simulink model "FlywheelSimscapeWithSensors"  (R2016a)
settings: Solver=VariableStepAuto  StartTime=0.0  StopTime=1000  RelTol=1e-3
undefined symbols (not defined in the file): sigbuilder_block
libraries: fl_lib x14, nesl_utility x8
settings Model: Creator=chiavazzo  LastModifiedBy=chiavazzo

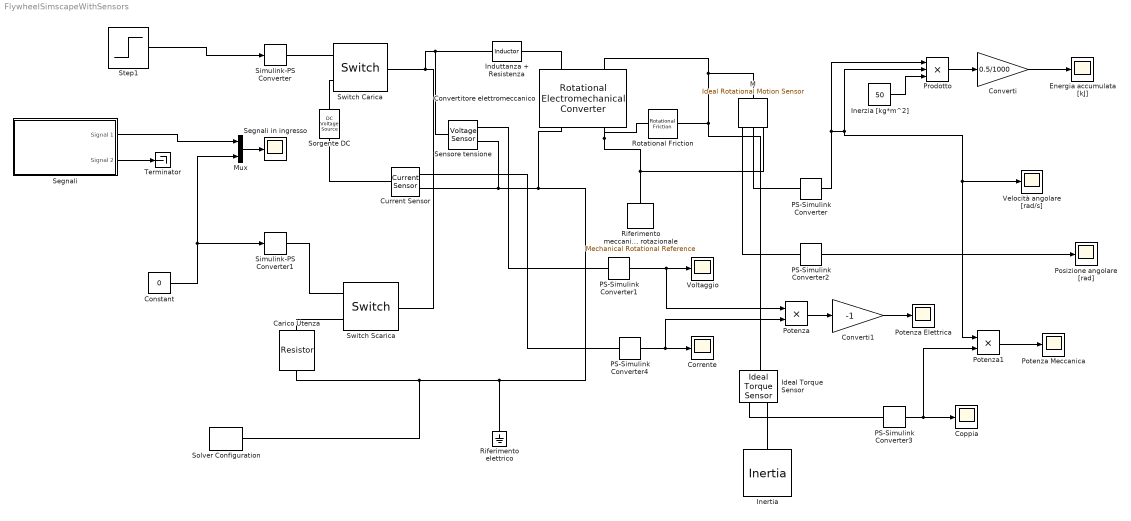
== system FlywheelSimscapeWithSensors ==
  " M" : fl_lib/Mechanical/Mechanical Sensors/Ideal Rotational Motion Sensor  offset=0 rad
  Carico Utenza : fl_lib/Electrical/Electrical Elements/Resistor  R=3 Ohm  i_specify=off  i_priority=None  i=0 A  v_specify=off  v_priority=None  v=0 V
  Constant : Constant  Value=0
  Converti : Gain  Gain=0.5/1000
  Converti1 : Gain  Gain=-1
  Convertitore elettromeccanico : fl_lib/Electrical/Electrical Elements/Rotational Electromechanical Converter  K=0.23 V/(rad/s)  i_specify=off  i_priority=None  i=0 A  v_specify=off  v_priority=None  v=0 V  t_specify=off  t_priority=None  t=0 N*m  w_specify=off  w_priority=None  w=0 rad/s
  Coppia : Scope
  Corrente : Scope
  Current Sensor : fl_lib/Electrical/Electrical Sensors/Current Sensor
  Energia accumulata [kJ] : Scope
  Ideal Torque Sensor : fl_lib/Mechanical/Mechanical Sensors/Ideal Torque Sensor
  Induttanza + Resistenza : fl_lib/Electrical/Electrical Elements/Inductor  l=5e-3 H  r=0.5 Ohm  g=1e-9 1/Ohm  i_specify=off  i_priority=None  i=0 A  v_specify=off  v_priority=None  v=0 V  i_L_specify=off  i_L_priority=High  i_L=0 A
  Inertia : fl_lib/Mechanical/Rotational Elements/Inertia  inertia=50 kg*m^2  w_specify=on  w_priority=High  w=0 rad/s  t_specify=off  t_priority=None  t=0 N*m
  Inerzia [kg*m^2] : Constant  Value=50
  Mux : Mux  Inputs=2
  PS-Simulink Converter{,1..4} (5 alike) : nesl_utility/PS-Simulink Converter  PhysicalDomain=network_engine_domain  SubClassName=ps_output  LeftPortType=input  RightPortType=output  PseudoPeriodic=off  Frequencies=[]  Unit=1  AffineConversion=off
  Posizione angolare [rad] : Scope
  Potenza : Product
  Potenza Elettrica : Scope
  Potenza Meccanica : Scope
  Potenza1 : Product
  "Prodotto " : Product  Inputs=3
  Riferimento meccanico rotazionale : fl_lib/Mechanical/Rotational Elements/Mechanical Rotational Reference
  Riferimento elettrico : fl_lib/Electrical/Electrical Elements/Electrical Reference
  Rotational Friction : fl_lib/Mechanical/Rotational Elements/Rotational Friction  brkwy_trq=25e-3 N*m  Col_trq=20e-3 N*m  visc_coef=0.01 N*m/(rad/s)  trans_coef=10 s/rad  vel_thr=1e-4 rad/s  w_specify=off  w_priority=None  w=0 rad/s  t_specify=off  t_priority=None  t=0 N*m
  Segnali : Subsystem  Tag=STV Subsys  LoadFcn=sigbuilder_block('load');  StartFcn=sigbuilder_block('start');  StopFcn=sigbuilder_block('stop');  ClipboardFcn=sigbuilder_block('clipboard');  mask(Sigbuilder block){}
      mask help: Simulink:masks:SigbuilderBlock_MD
      mask init:
      | if ~strcmp(get_param(bdroot(gcbh),'SimulationStatus'),'stopped') tuvar = sigbuilder_block('maskInit'); end
      settings: CopyFcn=sigbuilder_block('copy');  DeleteFcn=sigbuilder_block('delete');  ModelCloseFcn=sigbuilder_block('modelClose');  PreSaveFcn=sigbuilder_block('preSave');  PauseFcn=sigbuilder_block('pause');  ContinueFcn=sigbuilder_block('continue');  NameChangeFcn=sigbuilder_block('namechange');  OpenFcn=sigbuilder_block('open',[124.5 40.5 738 329.5 ]);  CloseFcn=sigbuilder_block('close');
      mask Display: plot(0, 0, 100, 100,[2, 2, 32, 32, 2], [68, 8, 8, 68, 68],[32, 2], [38, 38], [32, 19, 2],[53, 60, 44], [32, 17, 17, 2],[16, 16, 31, 31]);txt = getActiveGroup(gcbh);text(2, 100, txt,'verticalAlignment', 'top');
  Segnali in ingresso : Scope
  Sensore tensione : fl_lib/Electrical/Electrical Sensors/Voltage Sensor
  Simulink-PS Converter : nesl_utility/Simulink-PS Converter  PhysicalDomain=network_engine_domain  SubClassName=ps_input  LeftPortType=input  RightPortType=output  PseudoPeriodic=off  Frequencies=[]  NoiseDistribution=none  NoiseParameters=[]  Unit=1  AffineConversion=off  InputFiltering=off  SimscapeFilterOrder=1  InputFilterTimeConstant=0.001  UdotUserProvided=1
  Simulink-PS Converter1 : nesl_utility/Simulink-PS Converter  PhysicalDomain=network_engine_domain  SubClassName=ps_input  LeftPortType=input  RightPortType=output  PseudoPeriodic=off  Frequencies=[]  NoiseDistribution=none  NoiseParameters=[]  Unit=1  AffineConversion=off  InputFiltering=off  SimscapeFilterOrder=1  InputFilterTimeConstant=0.001  UdotUserProvided=1
  Solver Configuration : nesl_utility/Solver Configuration  PhysicalDomain=network_engine_domain  SubClassName=solver  LeftPortType=input  RightPortType=generic  Accelerate=off  Tones=[]  Harmonics=[]  SimulateNoise=off  Profile=off  UseLocalSampling=off  EnableSwitchedLinearOptims=on  FrequencyDomain=off  UseCCode=off  RelTol=0.001  AbsTol=1e-06  MinStep=1e-09  ToWorkspace=off  RevertToSquareIcSolve=off  NumHomotopyIterations=100  PhasorMode=off  PhasorModeNumHarmonics=1  OverrideAbsTol=off  DoDC=off  ResidualTolerance=1e-09  UseLocalSolver=on  LocalSolverChoice=NE_BACKWARD_EULER_ADVANCER  LocalSolverSampleTime=0.001  DoFixedCost=on  MaxNonlinIter=3  MaxModeIter=2  LinearAlgebra=Sparse  DelaysMemoryBudget=1024  AutomaticFiltering=on  FilteringTimeConstant=0.001
  Sorgente DC : fl_lib/Electrical/Electrical Sources/DC Voltage Source  v0=50 V
  Step1 : Step  Time=10  SampleTime=0
  Switch Carica : fl_lib/Electrical/Electrical Elements/Switch  R_closed=0.01 Ohm  G_open=1e-8 1/Ohm  Threshold=1e-3  i_specify=off  i_priority=None  i=0 A  v_specify=off  v_priority=None  v=0 V
  Switch Scarica : fl_lib/Electrical/Electrical Elements/Switch  R_closed=0.01 Ohm  G_open=1e-8 1/Ohm  Threshold=1e-3  i_specify=off  i_priority=None  i=0 A  v_specify=off  v_priority=None  v=0 V
  Terminator : Terminator
  Velocità angolare [rad/s] : Scope
  Voltaggio : Scope
  wires:
  PS-Simulink Converter/1 -> "Prodotto "/1, "Prodotto "/2, Potenza1/1, Velocità angolare [rad/s]/1
  PS-Simulink Converter2/1 -> Posizione angolare [rad]/1
  PS-Simulink Converter1/1 -> Potenza/1, Voltaggio/1
  "Prodotto "/1 -> Converti/1
  Inerzia [kg*m^2]/1 -> "Prodotto "/3
  Converti/1 -> Energia accumulata [kJ]/1
  Mux/1 -> Segnali in ingresso/1
  Constant/1 -> Mux/2, Simulink-PS Converter1/1
  Segnali/2(Signal 2) -> Terminator/1
  Step1/1 -> Simulink-PS Converter/1
  Segnali/1(Signal 1) -> Mux/1
  PS-Simulink Converter3/1 -> Potenza1/2, Coppia/1
  PS-Simulink Converter4/1 -> Potenza/2, Corrente/1
  Potenza/1 -> Converti1/1
  Potenza1/1 -> Potenza Meccanica/1
  Converti1/1 -> Potenza Elettrica/1
  connections:
  Induttanza + Resistenza/RConn1 -- Convertitore elettromeccanico/LConn1
  Convertitore elettromeccanico/RConn2 -- Rotational Friction/LConn1 -- " M"/RConn1 -- Riferimento meccanico rotazionale/LConn1
  " M"/RConn2 -- PS-Simulink Converter/LConn1
  " M"/RConn3 -- PS-Simulink Converter2/LConn1
  Sensore tensione/RConn1 -- PS-Simulink Converter1/LConn1
  Sorgente DC/LConn1 -- Switch Carica/RConn2
  Simulink-PS Converter/RConn1 -- Switch Carica/RConn1
  Carico Utenza/LConn1 -- Switch Scarica/RConn2
  Simulink-PS Converter1/RConn1 -- Switch Scarica/RConn1
  Solver Configuration/RConn1 -- Carico Utenza/RConn1 -- Riferimento elettrico/LConn1 -- Current Sensor/RConn2 -- Sensore tensione/RConn2 -- Convertitore elettromeccanico/RConn1
  Convertitore elettromeccanico/LConn2 -- Ideal Torque Sensor/LConn1 -- Rotational Friction/RConn1 -- " M"/LConn1
  Switch Carica/LConn1 -- Switch Scarica/LConn1 -- Sensore tensione/LConn1 -- Induttanza + Resistenza/LConn1
  PS-Simulink Converter4/LConn1 -- Current Sensor/RConn1
  Ideal Torque Sensor/RConn1 -- Inertia/LConn1
  Ideal Torque Sensor/RConn2 -- PS-Simulink Converter3/LConn1
  Current Sensor/LConn1 -- Sorgente DC/RConn1

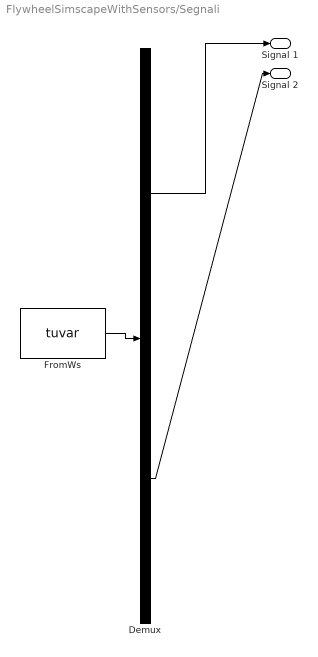
== system FlywheelSimscapeWithSensors/Segnali ==
  Demux : Demux  Tag=STV Demux  Outputs=2
  FromWs : FromWorkspace  Tag=STV FromWs  VariableName=tuvar  SampleTime=0
      SigBuilderData=|
      | common.afterFinalStr = 'Extrapolate'
      | common.sampleTime = 0
      | dataSet.timeRange = [0 15]
      | dataSet.name = 'Group 1'
      | sbobj.Groups.Name = 'Group 1'
      | sbobj.Groups.Signals(1).Name = 'Signal 1'
      | sbobj.Groups.Signals(1).XData = [0 4 6 6 15]
      | sbobj.Groups.Signals(1).YData = [1 1 1 0 0]
      | sbobj.Groups.Signals(2).Name = 'Signal 2'
      | sbobj.Groups.Signals(2).XData = [0 1 1.5 2 2.5 3 3.5 4 4.5 5 5.5 6 6.5 7 7.5 8 8.5 9 9.5 10 10 11 11.5 12 12.5 14.5 14.5 15]
      | sbobj.Groups.Signals(2).YData = [0 1.22464679915e-16 0 0 0 1.22464679915e-16 0 0 0 1.22464679915e-16 0 0 0 1.22464679915e-16 0 0 0 1.22464679915e-16 0 0 1 1 1 1 1 1 0 0]
      | sbobj.Groups.TimeRange = [0 15]
  Signal 1 : Outport  Tag=STV Outport
  Signal 2 : Outport  Tag=STV Outport  Port=2
  wires:
  Demux/1 -> Signal 1/1
  FromWs/1 -> Demux/1
  Demux/2 -> Signal 2/1
